simulink model "robusni_FPD_regulacija_nelin_sim"  (R2020a)
settings: Solver=ode3  StartTime=0.0  StopTime=tfin  FixedStep=1e-3  RelTol=1e-3
values from neighbouring files (symbols this model uses):
  derivative_e_lower_limit = -7.8663    [FPD_regulacija_nelin_sim_matlab.m]    (also in odredjivanje_granica_varijabli.m = -derivative_S_upper_limit; robusni_FPD_regulacija_nelin_sim_matlab.m)
  derivative_e_upper_limit = 7.8663    [FPD_regulacija_nelin_sim_matlab.m]    (also in odredjivanje_granica_varijabli.m = -derivative_S_lower_limit; robusni_FPD_regulacija_nelin_sim_matlab.m)
  disturb_X = 0.2*Xe    (= 0.978133730754)    [FPD_regulacija_nelin_sim_matlab.m]    (also in robusni_FPD_regulacija_nelin_sim_matlab.m)
  disturb_X_time = 5    [FPD_regulacija_nelin_sim_matlab.m]    (also in robusni_FPD_regulacija_nelin_sim_matlab.m)
  F_lower_limit = 0    [FPD_regulacija_nelin_sim_matlab.m]    (also in odredjivanje_granica_varijabli.m; robusni_FPD_regulacija_nelin_sim_matlab.m)
  F_upper_limit = Fe + 1e-3*Fe    (= 3.21211951185)    [FPD_regulacija_nelin_sim_matlab.m]    (also in odredjivanje_granica_varijabli.m = 3.2121089; robusni_FPD_regulacija_nelin_sim_matlab.m)
  K1 = 0.0300    (= 0.03)    [FPD_regulacija_nelin_sim_matlab.m]    (also in odredjivanje_granica_varijabli.m; robusni_FPD_regulacija_nelin_sim_matlab.m)
  K2 = 0.5000    (= 0.5)    [FPD_regulacija_nelin_sim_matlab.m]    (also in odredjivanje_granica_varijabli.m; robusni_FPD_regulacija_nelin_sim_matlab.m)
  mi0 = mie    (= 0.802227650313)    [FPD_regulacija_nelin_sim_matlab.m]    (also in robusni_FPD_regulacija_nelin_sim_matlab.m)
  mi_max = 1    [FPD_regulacija_nelin_sim_matlab.m]    (also in odredjivanje_granica_varijabli.m; robusni_FPD_regulacija_nelin_sim_matlab.m)
  S_step1 = delta    (= 0)    [FPD_regulacija_nelin_sim_matlab.m]    (also in robusni_FPD_regulacija_nelin_sim_matlab.m)
  S_step2 = delta    (= 0)    [FPD_regulacija_nelin_sim_matlab.m]    (also in robusni_FPD_regulacija_nelin_sim_matlab.m)
  S_time_step1 = 2    [FPD_regulacija_nelin_sim_matlab.m]    (also in robusni_FPD_regulacija_nelin_sim_matlab.m = 20)
  S_time_step2 = 40    [FPD_regulacija_nelin_sim_matlab.m]    (also in robusni_FPD_regulacija_nelin_sim_matlab.m = 50)
  Se = 0.218662692463450    (= 0.218662692463)    [FPD_regulacija_nelin_sim_matlab.m]    (also in odredjivanje_granica_varijabli.m = 0.2187; robusni_FPD_regulacija_nelin_sim_matlab.m)
  SF = 10.0000    (= 10)    [FPD_regulacija_nelin_sim_matlab.m]    (also in odredjivanje_granica_varijabli.m; robusni_FPD_regulacija_nelin_sim_matlab.m)
  std_noise = 1e-5*Se    (= 2.18662692463e-06)    [FPD_regulacija_nelin_sim_matlab.m]    (also in robusni_FPD_regulacija_nelin_sim_matlab.m = 0)
  V = 4.0000    (= 4)    [FPD_regulacija_nelin_sim_matlab.m]    (also in odredjivanje_granica_varijabli.m; robusni_FPD_regulacija_nelin_sim_matlab.m)
  x10 = Xe    (= 4.89066865377)    [FPD_regulacija_nelin_sim_matlab.m]    (also in odredjivanje_granica_varijabli.m = 5; robusni_FPD_regulacija_nelin_sim_matlab.m)
  x20 = Se    (= 0.218662692463)    [FPD_regulacija_nelin_sim_matlab.m]    (also in odredjivanje_granica_varijabli.m = 0; robusni_FPD_regulacija_nelin_sim_matlab.m)
  Y = 0.5000    (= 0.5)    [FPD_regulacija_nelin_sim_matlab.m]    (also in odredjivanje_granica_varijabli.m; robusni_FPD_regulacija_nelin_sim_matlab.m)
  Y1 = Y - 0.2*Y    (= 0.4)    [robusni_FPD_regulacija_nelin_sim_matlab.m]
  Y2 = Y - 0.1*Y    (= 0.45)    [robusni_FPD_regulacija_nelin_sim_matlab.m]
  Y3 = Y + 0.1*Y    (= 0.55)    [robusni_FPD_regulacija_nelin_sim_matlab.m]
  Y4 = Y + 0.2*Y    (= 0.6)    [robusni_FPD_regulacija_nelin_sim_matlab.m]
undefined symbols (not defined in the file or in its folder): magnitude
libraries: fuzblock x5
settings Model: Creator=anaMceranic  LastModifiedBy=anaMceranic
settings DataIOCC: ReturnWorkspaceOutputs=off

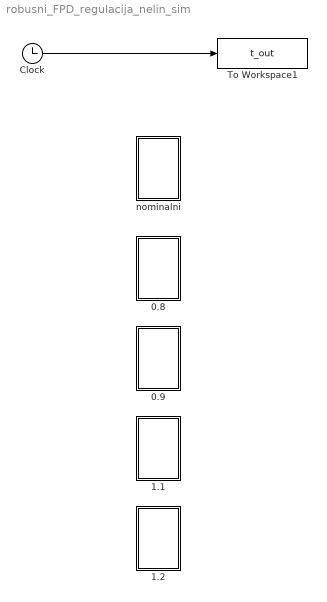
== system robusni_FPD_regulacija_nelin_sim ==
  0.8 : Subsystem
  0.9 : Subsystem
  1.1 : Subsystem
  1.2 : Subsystem
  Clock : Clock
  To Workspace1 : ToWorkspace  VariableName=t_out  SampleTime=-1
  nominalni : Subsystem
  wires:
  Clock/1 -> To Workspace1/1

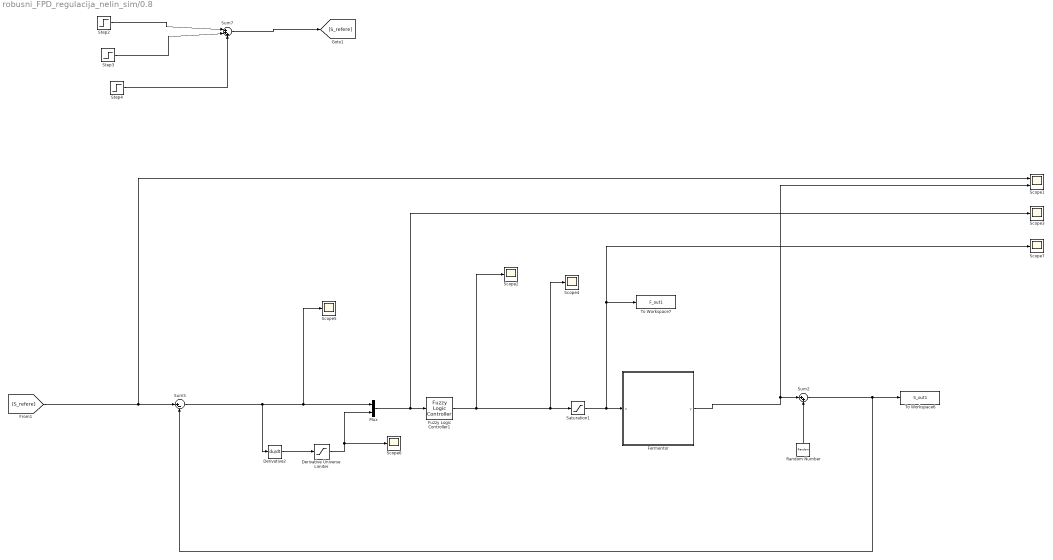
== system robusni_FPD_regulacija_nelin_sim/0.8 ==
  Derivative Universe Limiter : Saturate  UpperLimit=derivative_e_upper_limit  LowerLimit=derivative_e_lower_limit
  Derivative2 : Derivative
  Fermentor : Subsystem
  Fuzzy Logic Controller1 : fuzblock/Fuzzy Logic  Controller  FIS=FLC  OutputSampleNumber=101  DataType=double  FuzzifiedInputs=off  RuleFiringStrengths=off  RuleOutputs=off  AggregatedOutputs=off  SimulateUsing=Interpreted execution  OutOfRangeInputValueMessage=warning  NoRuleFiredMessage=warning  EmptyOutputFuzzySetMessage=warning
  Mux : Mux  Inputs=2
  Random Number : RandomNumber  Variance=std_noise  SampleTime=0.1
  Saturation1 : Saturate  UpperLimit=F_upper_limit  LowerLimit=F_lower_limit
  Scope1 : Scope  NumInputPorts=2
  Scope{2..7} (6 alike) : Scope
  Step2 : Step  Time=0  Before=Se  After=Se  SampleTime=0
  Step3 : Step  Time=S_time_step1  After=S_step1  SampleTime=0
  Step4 : Step  Time=S_time_step2  After=-S_step2  SampleTime=0
  Sum2 : Sum  Inputs=|++
  Sum5 : Sum  Inputs=|+-
  Sum7 : Sum  Inputs=|+++
  To Workspace6 : ToWorkspace  VariableName=S_out1  SampleTime=-1
  To Workspace7 : ToWorkspace  VariableName=F_out1  SampleTime=-1
  wires:
  Fermentor/1(y) -> Sum2/1, Scope1/2
  Saturation1/1 -> Fermentor/1(u), To Workspace7/1, Scope7/1
  Sum5/1 -> Mux/1, Scope5/1, Derivative2/1
  Mux/1 -> Scope3/1, Fuzzy Logic Controller1/1
  Derivative Universe Limiter/1 -> Mux/2, Scope6/1
  Sum2/1 -> To Workspace6/1, Sum5/2
  [S_refere] -> Sum5/1, Scope1/1
  Random Number/1 -> Sum2/2
  Derivative2/1 -> Derivative Universe Limiter/1
  Fuzzy Logic Controller1/1 -> Scope2/1, Saturation1/1, Scope4/1
  Step4/1 -> Sum7/3
  Step3/1 -> Sum7/2
  Sum7/1 -> [S_refere]
  Step2/1 -> Sum7/1

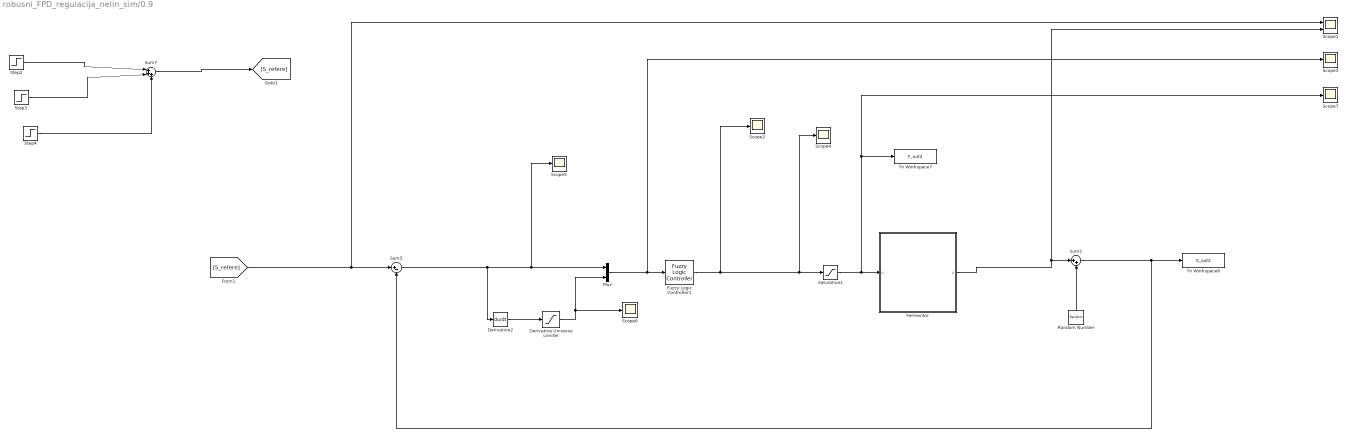
== system robusni_FPD_regulacija_nelin_sim/0.9 ==
  Derivative Universe Limiter : Saturate  UpperLimit=derivative_e_upper_limit  LowerLimit=derivative_e_lower_limit
  Derivative2 : Derivative
  Fermentor : Subsystem
  Fuzzy Logic Controller1 : fuzblock/Fuzzy Logic  Controller  FIS=FLC  OutputSampleNumber=101  DataType=double  FuzzifiedInputs=off  RuleFiringStrengths=off  RuleOutputs=off  AggregatedOutputs=off  SimulateUsing=Interpreted execution  OutOfRangeInputValueMessage=warning  NoRuleFiredMessage=warning  EmptyOutputFuzzySetMessage=warning
  Mux : Mux  Inputs=2
  Random Number : RandomNumber  Variance=std_noise  SampleTime=0.1
  Saturation1 : Saturate  UpperLimit=F_upper_limit  LowerLimit=F_lower_limit
  Scope1 : Scope  NumInputPorts=2
  Scope{2..7} (6 alike) : Scope
  Step2 : Step  Time=0  Before=Se  After=Se  SampleTime=0
  Step3 : Step  Time=S_time_step1  After=S_step1  SampleTime=0
  Step4 : Step  Time=S_time_step2  After=-S_step2  SampleTime=0
  Sum2 : Sum  Inputs=|++
  Sum5 : Sum  Inputs=|+-
  Sum7 : Sum  Inputs=|+++
  To Workspace6 : ToWorkspace  VariableName=S_out2  SampleTime=-1
  To Workspace7 : ToWorkspace  VariableName=F_out2  SampleTime=-1
  wires:
  Fuzzy Logic Controller1/1 -> Scope4/1, Saturation1/1, Scope2/1
  Derivative2/1 -> Derivative Universe Limiter/1
  Random Number/1 -> Sum2/2
  [S_refere] -> Scope1/1, Sum5/1
  Sum2/1 -> Sum5/2, To Workspace6/1
  Derivative Universe Limiter/1 -> Scope6/1, Mux/2
  Mux/1 -> Fuzzy Logic Controller1/1, Scope3/1
  Sum5/1 -> Derivative2/1, Scope5/1, Mux/1
  Saturation1/1 -> Scope7/1, To Workspace7/1, Fermentor/1(u)
  Fermentor/1(y) -> Scope1/2, Sum2/1
  Step4/1 -> Sum7/3
  Step3/1 -> Sum7/2
  Sum7/1 -> [S_refere]
  Step2/1 -> Sum7/1

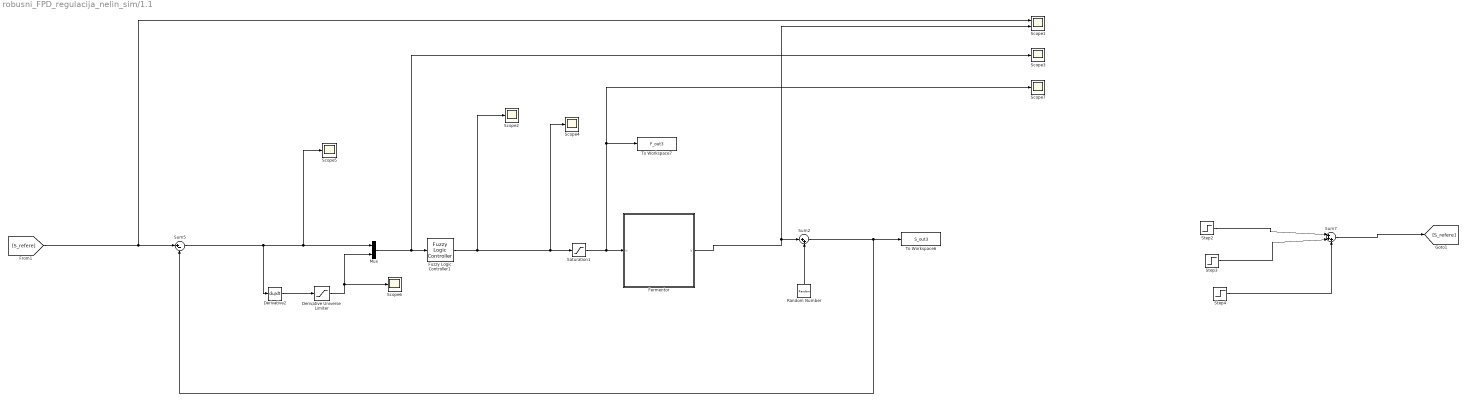
== system robusni_FPD_regulacija_nelin_sim/1.1 ==
  Derivative Universe Limiter : Saturate  UpperLimit=derivative_e_upper_limit  LowerLimit=derivative_e_lower_limit
  Derivative2 : Derivative
  Fermentor : Subsystem
  Fuzzy Logic Controller1 : fuzblock/Fuzzy Logic  Controller  FIS=FLC  OutputSampleNumber=101  DataType=double  FuzzifiedInputs=off  RuleFiringStrengths=off  RuleOutputs=off  AggregatedOutputs=off  SimulateUsing=Interpreted execution  OutOfRangeInputValueMessage=warning  NoRuleFiredMessage=warning  EmptyOutputFuzzySetMessage=warning
  Mux : Mux  Inputs=2
  Random Number : RandomNumber  Variance=std_noise  SampleTime=0.1
  Saturation1 : Saturate  UpperLimit=F_upper_limit  LowerLimit=F_lower_limit
  Scope1 : Scope  NumInputPorts=2
  Scope{2..7} (6 alike) : Scope
  Step2 : Step  Time=0  Before=Se  After=Se  SampleTime=0
  Step3 : Step  Time=S_time_step1  After=S_step1  SampleTime=0
  Step4 : Step  Time=S_time_step2  After=-S_step2  SampleTime=0
  Sum2 : Sum  Inputs=|++
  Sum5 : Sum  Inputs=|+-
  Sum7 : Sum  Inputs=|+++
  To Workspace6 : ToWorkspace  VariableName=S_out3  SampleTime=-1
  To Workspace7 : ToWorkspace  VariableName=F_out3  SampleTime=-1
  wires:
  Fermentor/1(y) -> Sum2/1, Scope1/2
  Saturation1/1 -> Fermentor/1(u), To Workspace7/1, Scope7/1
  Sum5/1 -> Mux/1, Scope5/1, Derivative2/1
  Mux/1 -> Scope3/1, Fuzzy Logic Controller1/1
  Derivative Universe Limiter/1 -> Mux/2, Scope6/1
  Sum2/1 -> To Workspace6/1, Sum5/2
  [S_refere] -> Sum5/1, Scope1/1
  Random Number/1 -> Sum2/2
  Derivative2/1 -> Derivative Universe Limiter/1
  Fuzzy Logic Controller1/1 -> Scope2/1, Saturation1/1, Scope4/1
  Step4/1 -> Sum7/3
  Step3/1 -> Sum7/2
  Sum7/1 -> [S_refere]
  Step2/1 -> Sum7/1

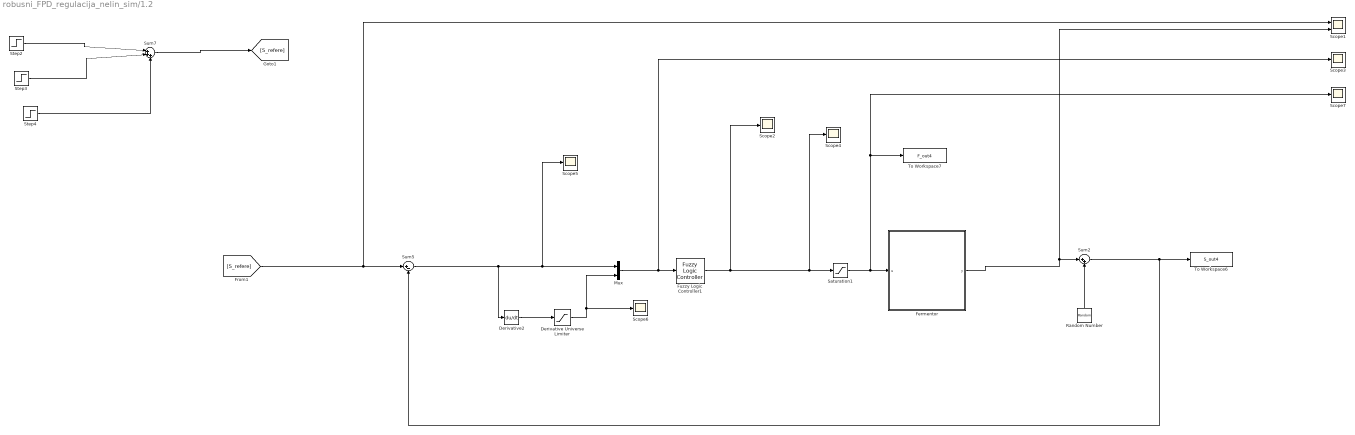
== system robusni_FPD_regulacija_nelin_sim/1.2 ==
  Derivative Universe Limiter : Saturate  UpperLimit=derivative_e_upper_limit  LowerLimit=derivative_e_lower_limit
  Derivative2 : Derivative
  Fermentor : Subsystem
  Fuzzy Logic Controller1 : fuzblock/Fuzzy Logic  Controller  FIS=FLC  OutputSampleNumber=101  DataType=double  FuzzifiedInputs=off  RuleFiringStrengths=off  RuleOutputs=off  AggregatedOutputs=off  SimulateUsing=Interpreted execution  OutOfRangeInputValueMessage=warning  NoRuleFiredMessage=warning  EmptyOutputFuzzySetMessage=warning
  Mux : Mux  Inputs=2
  Random Number : RandomNumber  Variance=std_noise  SampleTime=0.1
  Saturation1 : Saturate  UpperLimit=F_upper_limit  LowerLimit=F_lower_limit
  Scope1 : Scope  NumInputPorts=2
  Scope{2..7} (6 alike) : Scope
  Step2 : Step  Time=0  Before=Se  After=Se  SampleTime=0
  Step3 : Step  Time=S_time_step1  After=S_step1  SampleTime=0
  Step4 : Step  Time=S_time_step2  After=-S_step2  SampleTime=0
  Sum2 : Sum  Inputs=|++
  Sum5 : Sum  Inputs=|+-
  Sum7 : Sum  Inputs=|+++
  To Workspace6 : ToWorkspace  VariableName=S_out4  SampleTime=-1
  To Workspace7 : ToWorkspace  VariableName=F_out4  SampleTime=-1
  wires:
  Fuzzy Logic Controller1/1 -> Scope4/1, Saturation1/1, Scope2/1
  Derivative2/1 -> Derivative Universe Limiter/1
  Random Number/1 -> Sum2/2
  [S_refere] -> Scope1/1, Sum5/1
  Sum2/1 -> Sum5/2, To Workspace6/1
  Derivative Universe Limiter/1 -> Scope6/1, Mux/2
  Mux/1 -> Fuzzy Logic Controller1/1, Scope3/1
  Sum5/1 -> Derivative2/1, Scope5/1, Mux/1
  Saturation1/1 -> Scope7/1, To Workspace7/1, Fermentor/1(u)
  Fermentor/1(y) -> Scope1/2, Sum2/1
  Step4/1 -> Sum7/3
  Step3/1 -> Sum7/2
  Sum7/1 -> [S_refere]
  Step2/1 -> Sum7/1

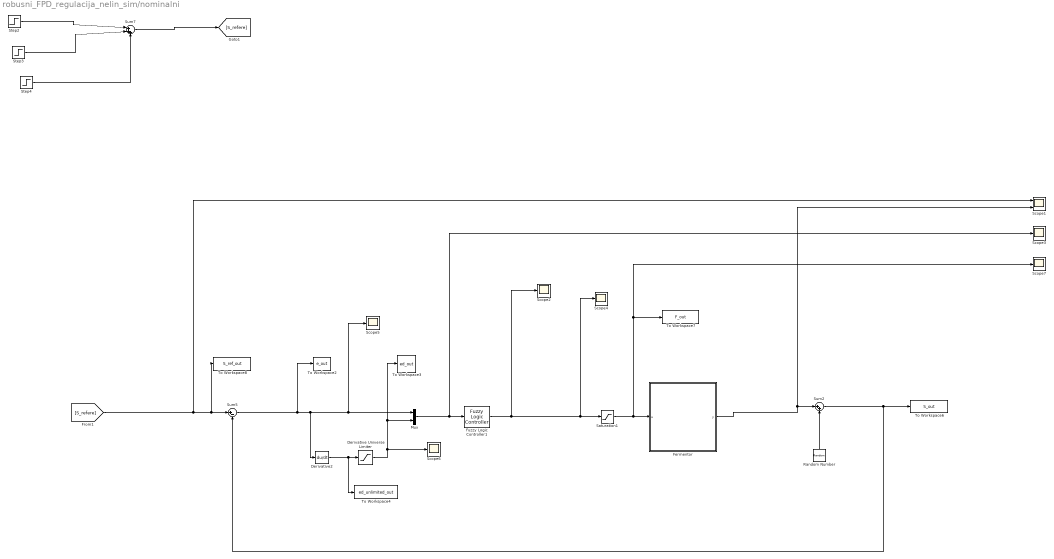
== system robusni_FPD_regulacija_nelin_sim/nominalni ==
  Derivative Universe Limiter : Saturate  UpperLimit=derivative_e_upper_limit  LowerLimit=derivative_e_lower_limit
  Derivative2 : Derivative
  Fermentor : Subsystem
  Fuzzy Logic Controller1 : fuzblock/Fuzzy Logic  Controller  FIS=FLC  OutputSampleNumber=101  DataType=double  FuzzifiedInputs=off  RuleFiringStrengths=off  RuleOutputs=off  AggregatedOutputs=off  SimulateUsing=Interpreted execution  OutOfRangeInputValueMessage=warning  NoRuleFiredMessage=warning  EmptyOutputFuzzySetMessage=warning
  Mux : Mux  Inputs=2
  Random Number : RandomNumber  Variance=std_noise  SampleTime=0.1
  Saturation1 : Saturate  UpperLimit=F_upper_limit  LowerLimit=F_lower_limit
  Scope1 : Scope  NumInputPorts=2
  Scope{2..7} (6 alike) : Scope
  Step2 : Step  Time=0  Before=Se  After=Se  SampleTime=0
  Step3 : Step  Time=S_time_step1  After=S_step1  SampleTime=0
  Step4 : Step  Time=S_time_step2  After=-S_step2  SampleTime=0
  Sum2 : Sum  Inputs=|++
  Sum5 : Sum  Inputs=|+-
  Sum7 : Sum  Inputs=|+++
  To Workspace2 : ToWorkspace  VariableName=e_out  SampleTime=-1
  To Workspace3 : ToWorkspace  VariableName=ed_out  SampleTime=-1
  To Workspace4 : ToWorkspace  VariableName=ed_unlimited_out  SampleTime=-1
  To Workspace6 : ToWorkspace  VariableName=S_out  SampleTime=-1
  To Workspace7 : ToWorkspace  VariableName=F_out  SampleTime=-1
  To Workspace8 : ToWorkspace  VariableName=S_ref_out  SampleTime=-1
  wires:
  Fuzzy Logic Controller1/1 -> Scope4/1, Saturation1/1, Scope2/1
  Derivative2/1 -> Derivative Universe Limiter/1, To Workspace4/1
  Random Number/1 -> Sum2/2
  [S_refere] -> Scope1/1, To Workspace8/1, Sum5/1
  Sum2/1 -> Sum5/2, To Workspace6/1
  Derivative Universe Limiter/1 -> Scope6/1, Mux/2, To Workspace3/1
  Mux/1 -> Fuzzy Logic Controller1/1, Scope3/1
  Sum5/1 -> Derivative2/1, Scope5/1, Mux/1, To Workspace2/1
  Saturation1/1 -> Scope7/1, To Workspace7/1, Fermentor/1(u)
  Fermentor/1(y) -> Scope1/2, Sum2/1
  Step4/1 -> Sum7/3
  Step3/1 -> Sum7/2
  Sum7/1 -> [S_refere]
  Step2/1 -> Sum7/1

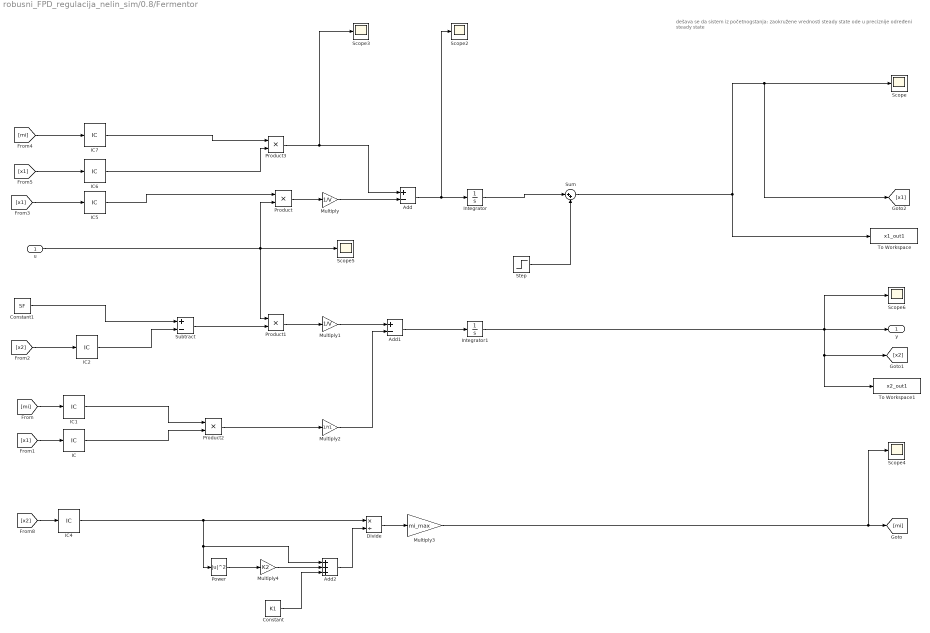
== system robusni_FPD_regulacija_nelin_sim/0.8/Fermentor ==
  note: dešava se da sistem iz početnogstanja: zaokružene vrednosti steady state
      | ode u preciznije određeni steady state
  u : Inport
  Add : Sum  Inputs=+-
  Add1 : Sum  Inputs=+-
  Add2 : Sum  Inputs=+++
  Constant : Constant  Value=K1
  Constant1 : Constant  Value=SF
  Divide : Product  Inputs=*/
  IC : InitialCondition  Value=x10
  IC1 : InitialCondition  Value=mi0
  IC2 : InitialCondition  Value=x20
  IC4 : InitialCondition  Value=x20
  IC5 : InitialCondition  Value=x10
  IC6 : InitialCondition  Value=x10
  IC7 : InitialCondition  Value=mi0
  Integrator : Integrator  InitialCondition=x10
  Integrator1 : Integrator  InitialCondition=x20
  Multiply : Gain  Gain=1/V
  Multiply1 : Gain  Gain=1/V
  Multiply2 : Gain  Gain=1/Y1
  Multiply3 : Gain  Gain=mi_max
  Multiply4 : Gain  Gain=K2
  Power : Math  Operator=magnitude^2  SaturateOnIntegerOverflow=on
  Product{,1..3} (4 alike) : Product
  Scope{,2..6} (6 alike) : Scope
  Step : Step  Time=disturb_X_time  After=disturb_X  SampleTime=0
  Subtract : Sum  Inputs=+-
  Sum : Sum  Inputs=|++
  To Workspace : ToWorkspace  VariableName=x1_out1  SampleTime=-1
  To Workspace1 : ToWorkspace  VariableName=x2_out1  SampleTime=-1
  y : Outport
  wires:
  Integrator/1 -> Sum/1
  Step/1 -> Sum/2
  Sum/1 -> [x1], Scope/1, To Workspace/1
  IC7/1 -> Product3/1
  IC6/1 -> Product3/2
  IC5/1 -> Product/1
  IC4/1 -> Power/1, Add2/1, Divide/1
  Constant1/1 -> Subtract/1
  IC2/1 -> Subtract/2
  IC1/1 -> Product2/1
  IC/1 -> Product2/2
  Integrator1/1 -> y/1, [x2], To Workspace1/1, Scope6/1
  Multiply3/1 -> Scope4/1, [mi]
  [mi] -> IC7/1
  Product/1 -> Multiply/1
  Add/1 -> Integrator/1, Scope2/1
  [x2] -> IC4/1
  Subtract/1 -> Product1/2
  Product1/1 -> Multiply1/1
  Multiply1/1 -> Add1/1
  [x1] -> IC5/1
  u/1 -> Scope5/1, Product1/1, Product/2
  Product3/1 -> Add/1, Scope3/1
  Divide/1 -> Multiply3/1
  Multiply2/1 -> Add1/2
  Add1/1 -> Integrator1/1
  [x2] -> IC2/1
  Power/1 -> Multiply4/1
  [mi] -> IC1/1
  Multiply4/1 -> Add2/2
  [x1] -> IC6/1
  Constant/1 -> Add2/3
  Add2/1 -> Divide/2
  Multiply/1 -> Add/2
  Product2/1 -> Multiply2/1
  [x1] -> IC/1

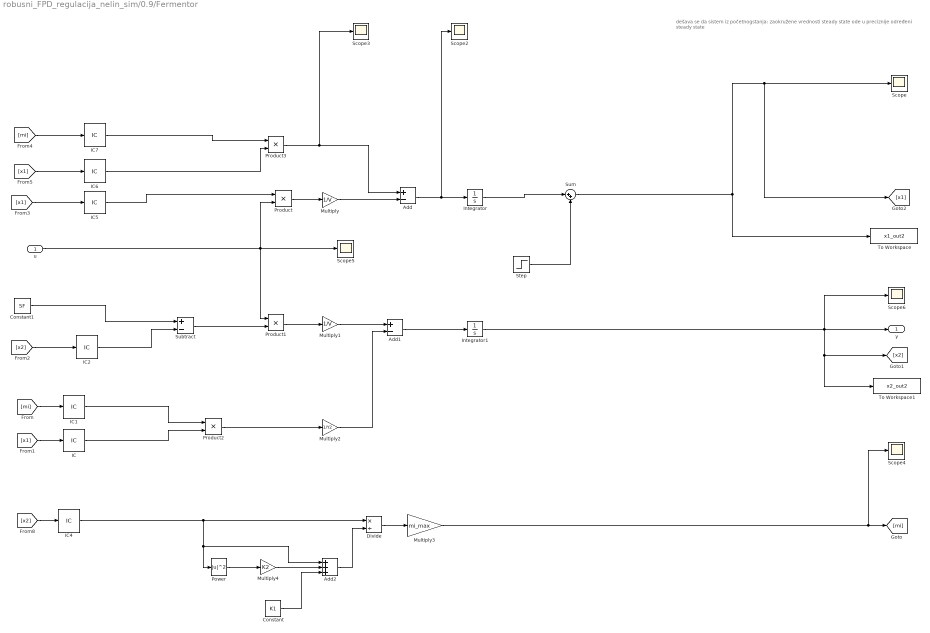
== system robusni_FPD_regulacija_nelin_sim/0.9/Fermentor ==
  note: dešava se da sistem iz početnogstanja: zaokružene vrednosti steady state
      | ode u preciznije određeni steady state
  u : Inport
  Add : Sum  Inputs=+-
  Add1 : Sum  Inputs=+-
  Add2 : Sum  Inputs=+++
  Constant : Constant  Value=K1
  Constant1 : Constant  Value=SF
  Divide : Product  Inputs=*/
  IC : InitialCondition  Value=x10
  IC1 : InitialCondition  Value=mi0
  IC2 : InitialCondition  Value=x20
  IC4 : InitialCondition  Value=x20
  IC5 : InitialCondition  Value=x10
  IC6 : InitialCondition  Value=x10
  IC7 : InitialCondition  Value=mi0
  Integrator : Integrator  InitialCondition=x10
  Integrator1 : Integrator  InitialCondition=x20
  Multiply : Gain  Gain=1/V
  Multiply1 : Gain  Gain=1/V
  Multiply2 : Gain  Gain=1/Y2
  Multiply3 : Gain  Gain=mi_max
  Multiply4 : Gain  Gain=K2
  Power : Math  Operator=magnitude^2  SaturateOnIntegerOverflow=on
  Product{,1..3} (4 alike) : Product
  Scope{,2..6} (6 alike) : Scope
  Step : Step  Time=disturb_X_time  After=disturb_X  SampleTime=0
  Subtract : Sum  Inputs=+-
  Sum : Sum  Inputs=|++
  To Workspace : ToWorkspace  VariableName=x1_out2  SampleTime=-1
  To Workspace1 : ToWorkspace  VariableName=x2_out2  SampleTime=-1
  y : Outport
  wires:
  [x1] -> IC/1
  Product2/1 -> Multiply2/1
  Multiply/1 -> Add/2
  Add2/1 -> Divide/2
  Constant/1 -> Add2/3
  [x1] -> IC6/1
  Multiply4/1 -> Add2/2
  [mi] -> IC1/1
  Power/1 -> Multiply4/1
  [x2] -> IC2/1
  Add1/1 -> Integrator1/1
  Multiply2/1 -> Add1/2
  Divide/1 -> Multiply3/1
  Product3/1 -> Scope3/1, Add/1
  u/1 -> Product/2, Product1/1, Scope5/1
  [x1] -> IC5/1
  Multiply1/1 -> Add1/1
  Product1/1 -> Multiply1/1
  Subtract/1 -> Product1/2
  [x2] -> IC4/1
  Add/1 -> Scope2/1, Integrator/1
  Product/1 -> Multiply/1
  [mi] -> IC7/1
  Multiply3/1 -> [mi], Scope4/1
  Integrator1/1 -> Scope6/1, To Workspace1/1, [x2], y/1
  IC/1 -> Product2/2
  IC1/1 -> Product2/1
  IC2/1 -> Subtract/2
  Constant1/1 -> Subtract/1
  IC4/1 -> Divide/1, Add2/1, Power/1
  IC5/1 -> Product/1
  IC6/1 -> Product3/2
  IC7/1 -> Product3/1
  Sum/1 -> To Workspace/1, Scope/1, [x1]
  Step/1 -> Sum/2
  Integrator/1 -> Sum/1

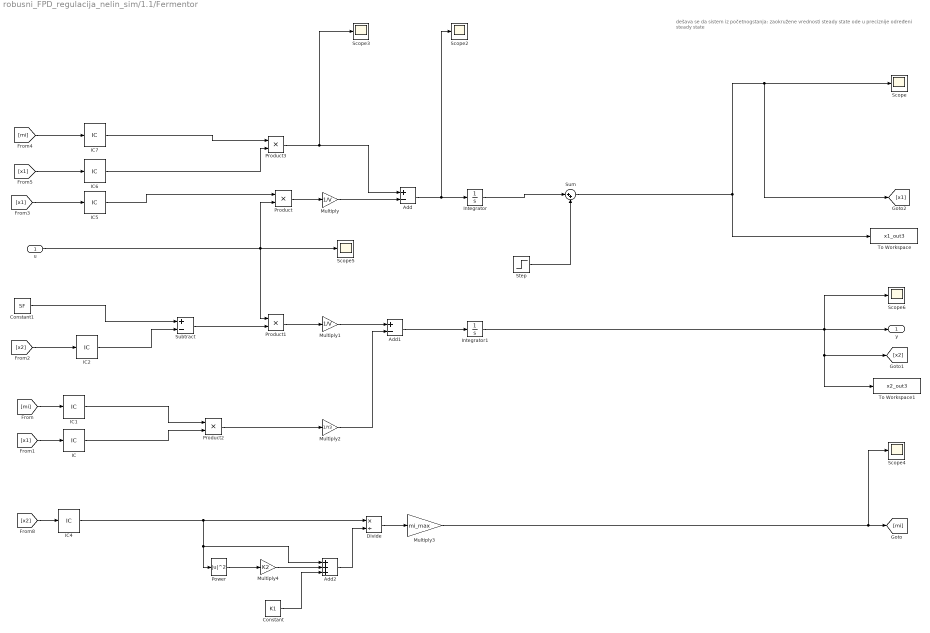
== system robusni_FPD_regulacija_nelin_sim/1.1/Fermentor ==
  note: dešava se da sistem iz početnogstanja: zaokružene vrednosti steady state
      | ode u preciznije određeni steady state
  u : Inport
  Add : Sum  Inputs=+-
  Add1 : Sum  Inputs=+-
  Add2 : Sum  Inputs=+++
  Constant : Constant  Value=K1
  Constant1 : Constant  Value=SF
  Divide : Product  Inputs=*/
  IC : InitialCondition  Value=x10
  IC1 : InitialCondition  Value=mi0
  IC2 : InitialCondition  Value=x20
  IC4 : InitialCondition  Value=x20
  IC5 : InitialCondition  Value=x10
  IC6 : InitialCondition  Value=x10
  IC7 : InitialCondition  Value=mi0
  Integrator : Integrator  InitialCondition=x10
  Integrator1 : Integrator  InitialCondition=x20
  Multiply : Gain  Gain=1/V
  Multiply1 : Gain  Gain=1/V
  Multiply2 : Gain  Gain=1/Y3
  Multiply3 : Gain  Gain=mi_max
  Multiply4 : Gain  Gain=K2
  Power : Math  Operator=magnitude^2  SaturateOnIntegerOverflow=on
  Product{,1..3} (4 alike) : Product
  Scope{,2..6} (6 alike) : Scope
  Step : Step  Time=disturb_X_time  After=disturb_X  SampleTime=0
  Subtract : Sum  Inputs=+-
  Sum : Sum  Inputs=|++
  To Workspace : ToWorkspace  VariableName=x1_out3  SampleTime=-1
  To Workspace1 : ToWorkspace  VariableName=x2_out3  SampleTime=-1
  y : Outport
  wires:
  Integrator/1 -> Sum/1
  Step/1 -> Sum/2
  Sum/1 -> [x1], Scope/1, To Workspace/1
  IC7/1 -> Product3/1
  IC6/1 -> Product3/2
  IC5/1 -> Product/1
  IC4/1 -> Power/1, Add2/1, Divide/1
  Constant1/1 -> Subtract/1
  IC2/1 -> Subtract/2
  IC1/1 -> Product2/1
  IC/1 -> Product2/2
  Integrator1/1 -> y/1, [x2], To Workspace1/1, Scope6/1
  Multiply3/1 -> Scope4/1, [mi]
  [mi] -> IC7/1
  Product/1 -> Multiply/1
  Add/1 -> Integrator/1, Scope2/1
  [x2] -> IC4/1
  Subtract/1 -> Product1/2
  Product1/1 -> Multiply1/1
  Multiply1/1 -> Add1/1
  [x1] -> IC5/1
  u/1 -> Scope5/1, Product1/1, Product/2
  Product3/1 -> Add/1, Scope3/1
  Divide/1 -> Multiply3/1
  Multiply2/1 -> Add1/2
  Add1/1 -> Integrator1/1
  [x2] -> IC2/1
  Power/1 -> Multiply4/1
  [mi] -> IC1/1
  Multiply4/1 -> Add2/2
  [x1] -> IC6/1
  Constant/1 -> Add2/3
  Add2/1 -> Divide/2
  Multiply/1 -> Add/2
  Product2/1 -> Multiply2/1
  [x1] -> IC/1

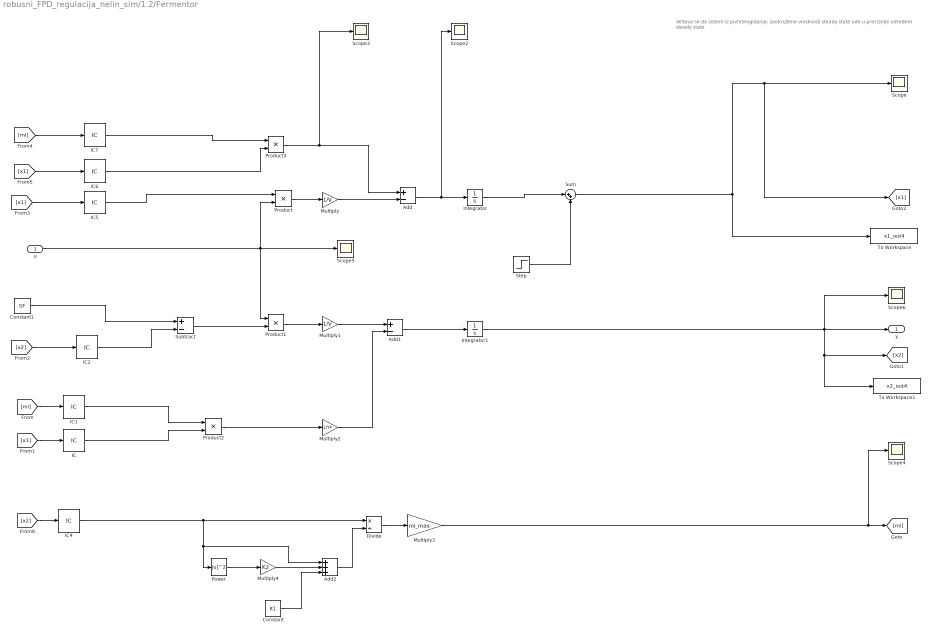
== system robusni_FPD_regulacija_nelin_sim/1.2/Fermentor ==
  note: dešava se da sistem iz početnogstanja: zaokružene vrednosti steady state
      | ode u preciznije određeni steady state
  u : Inport
  Add : Sum  Inputs=+-
  Add1 : Sum  Inputs=+-
  Add2 : Sum  Inputs=+++
  Constant : Constant  Value=K1
  Constant1 : Constant  Value=SF
  Divide : Product  Inputs=*/
  IC : InitialCondition  Value=x10
  IC1 : InitialCondition  Value=mi0
  IC2 : InitialCondition  Value=x20
  IC4 : InitialCondition  Value=x20
  IC5 : InitialCondition  Value=x10
  IC6 : InitialCondition  Value=x10
  IC7 : InitialCondition  Value=mi0
  Integrator : Integrator  InitialCondition=x10
  Integrator1 : Integrator  InitialCondition=x20
  Multiply : Gain  Gain=1/V
  Multiply1 : Gain  Gain=1/V
  Multiply2 : Gain  Gain=1/Y4
  Multiply3 : Gain  Gain=mi_max
  Multiply4 : Gain  Gain=K2
  Power : Math  Operator=magnitude^2  SaturateOnIntegerOverflow=on
  Product{,1..3} (4 alike) : Product
  Scope{,2..6} (6 alike) : Scope
  Step : Step  Time=disturb_X_time  After=disturb_X  SampleTime=0
  Subtract : Sum  Inputs=+-
  Sum : Sum  Inputs=|++
  To Workspace : ToWorkspace  VariableName=x1_out4  SampleTime=-1
  To Workspace1 : ToWorkspace  VariableName=x2_out4  SampleTime=-1
  y : Outport
  wires:
  [x1] -> IC/1
  Product2/1 -> Multiply2/1
  Multiply/1 -> Add/2
  Add2/1 -> Divide/2
  Constant/1 -> Add2/3
  [x1] -> IC6/1
  Multiply4/1 -> Add2/2
  [mi] -> IC1/1
  Power/1 -> Multiply4/1
  [x2] -> IC2/1
  Add1/1 -> Integrator1/1
  Multiply2/1 -> Add1/2
  Divide/1 -> Multiply3/1
  Product3/1 -> Scope3/1, Add/1
  u/1 -> Product/2, Product1/1, Scope5/1
  [x1] -> IC5/1
  Multiply1/1 -> Add1/1
  Product1/1 -> Multiply1/1
  Subtract/1 -> Product1/2
  [x2] -> IC4/1
  Add/1 -> Scope2/1, Integrator/1
  Product/1 -> Multiply/1
  [mi] -> IC7/1
  Multiply3/1 -> [mi], Scope4/1
  Integrator1/1 -> Scope6/1, To Workspace1/1, [x2], y/1
  IC/1 -> Product2/2
  IC1/1 -> Product2/1
  IC2/1 -> Subtract/2
  Constant1/1 -> Subtract/1
  IC4/1 -> Divide/1, Add2/1, Power/1
  IC5/1 -> Product/1
  IC6/1 -> Product3/2
  IC7/1 -> Product3/1
  Sum/1 -> To Workspace/1, Scope/1, [x1]
  Step/1 -> Sum/2
  Integrator/1 -> Sum/1

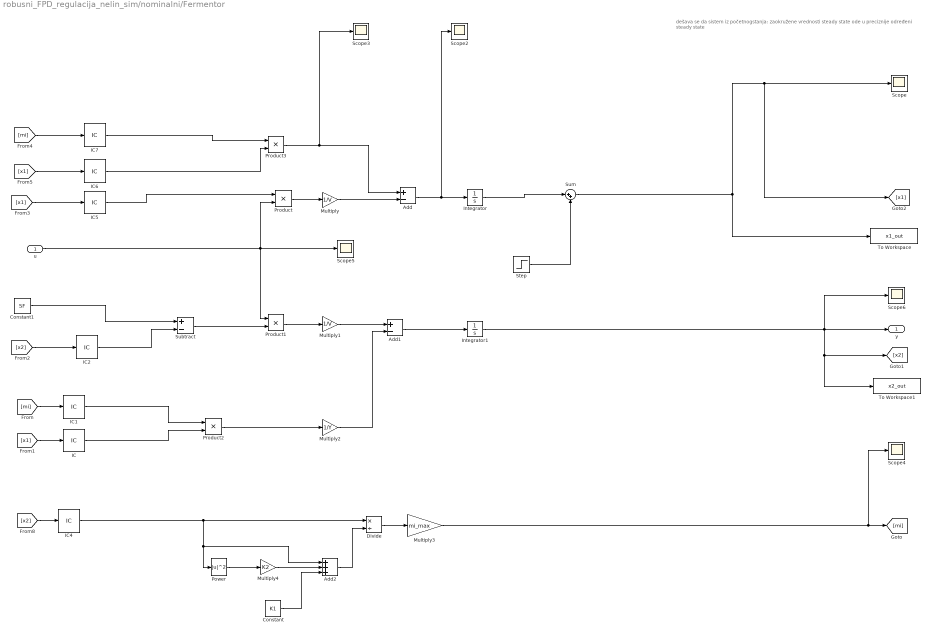
== system robusni_FPD_regulacija_nelin_sim/nominalni/Fermentor ==
  note: dešava se da sistem iz početnogstanja: zaokružene vrednosti steady state
      | ode u preciznije određeni steady state
  u : Inport
  Add : Sum  Inputs=+-
  Add1 : Sum  Inputs=+-
  Add2 : Sum  Inputs=+++
  Constant : Constant  Value=K1
  Constant1 : Constant  Value=SF
  Divide : Product  Inputs=*/
  IC : InitialCondition  Value=x10
  IC1 : InitialCondition  Value=mi0
  IC2 : InitialCondition  Value=x20
  IC4 : InitialCondition  Value=x20
  IC5 : InitialCondition  Value=x10
  IC6 : InitialCondition  Value=x10
  IC7 : InitialCondition  Value=mi0
  Integrator : Integrator  InitialCondition=x10
  Integrator1 : Integrator  InitialCondition=x20
  Multiply : Gain  Gain=1/V
  Multiply1 : Gain  Gain=1/V
  Multiply2 : Gain  Gain=1/Y
  Multiply3 : Gain  Gain=mi_max
  Multiply4 : Gain  Gain=K2
  Power : Math  Operator=magnitude^2  SaturateOnIntegerOverflow=on
  Product{,1..3} (4 alike) : Product
  Scope{,2..6} (6 alike) : Scope
  Step : Step  Time=disturb_X_time  After=disturb_X  SampleTime=0
  Subtract : Sum  Inputs=+-
  Sum : Sum  Inputs=|++
  To Workspace : ToWorkspace  VariableName=x1_out  SampleTime=-1
  To Workspace1 : ToWorkspace  VariableName=x2_out  SampleTime=-1
  y : Outport
  wires:
  [x1] -> IC/1
  Product2/1 -> Multiply2/1
  Multiply/1 -> Add/2
  Add2/1 -> Divide/2
  Constant/1 -> Add2/3
  [x1] -> IC6/1
  Multiply4/1 -> Add2/2
  [mi] -> IC1/1
  Power/1 -> Multiply4/1
  [x2] -> IC2/1
  Add1/1 -> Integrator1/1
  Multiply2/1 -> Add1/2
  Divide/1 -> Multiply3/1
  Product3/1 -> Scope3/1, Add/1
  u/1 -> Product/2, Product1/1, Scope5/1
  [x1] -> IC5/1
  Multiply1/1 -> Add1/1
  Product1/1 -> Multiply1/1
  Subtract/1 -> Product1/2
  [x2] -> IC4/1
  Add/1 -> Scope2/1, Integrator/1
  Product/1 -> Multiply/1
  [mi] -> IC7/1
  Multiply3/1 -> [mi], Scope4/1
  Integrator1/1 -> Scope6/1, To Workspace1/1, [x2], y/1
  IC/1 -> Product2/2
  IC1/1 -> Product2/1
  IC2/1 -> Subtract/2
  Constant1/1 -> Subtract/1
  IC4/1 -> Divide/1, Add2/1, Power/1
  IC5/1 -> Product/1
  IC6/1 -> Product3/2
  IC7/1 -> Product3/1
  Sum/1 -> To Workspace/1, Scope/1, [x1]
  Step/1 -> Sum/2
  Integrator/1 -> Sum/1
